simulink model "DC_current_phasor"  (R2016a)
settings: Solver=ode23t  StartTime=0.0  StopTime=2  MaxStep=1e-4  RelTol=1e-4  AbsTol=1e-4
undefined symbols (not defined in the file or in its folder): j, P
libraries: fl_lib x8, nesl_utility x8, pe_lib x3, ThreePhaseExamples_lib x1
Description:
  | Three-Phase Custom PMSM
  | 
  | This example shows a custom Simscape(TM) implementation of
  | a Permanent Magnet Synchronous Machine (PMSM). To view the
  | PMSM source code, double-click on the motor block and then
  | click on the hyperlink 'Source code'. This test circuit shows the
  | PMSM being used as a generator, the rectifier block converting
  | the induced AC back EMFs to a DC voltage which is in turn
  | applied to a resistive load.
  | 
  | 
  | 
  | Copyright 2008-2016 The MathWorks, Inc.
settings Model: Creator=MathWorks  LastModifiedBy=hbjo
settings DataIOCC: LimitDataPoints=on  SaveFormat=Array
settings DebuggingCC: UnderspecifiedInitializationDetection=Classic  MergeDetectMultiDrivingBlocksExec=none
settings HardwareCC: ProdBitPerPointer=32  ProdLargestAtomicFloat=None  ProdIntDivRoundTo=Undefined  ProdEndianess=Unspecified  ProdWordSize=32  ProdHWDeviceType=32-bit Generic
settings ModelReferenceCC: PropagateSignalLabelsOutOfModel=off
settings ConfigComp: CovModelRefEnable=Off  CovSFcnEnable=off
settings SimscapeCC: SimscapeLogDataHistory=50000

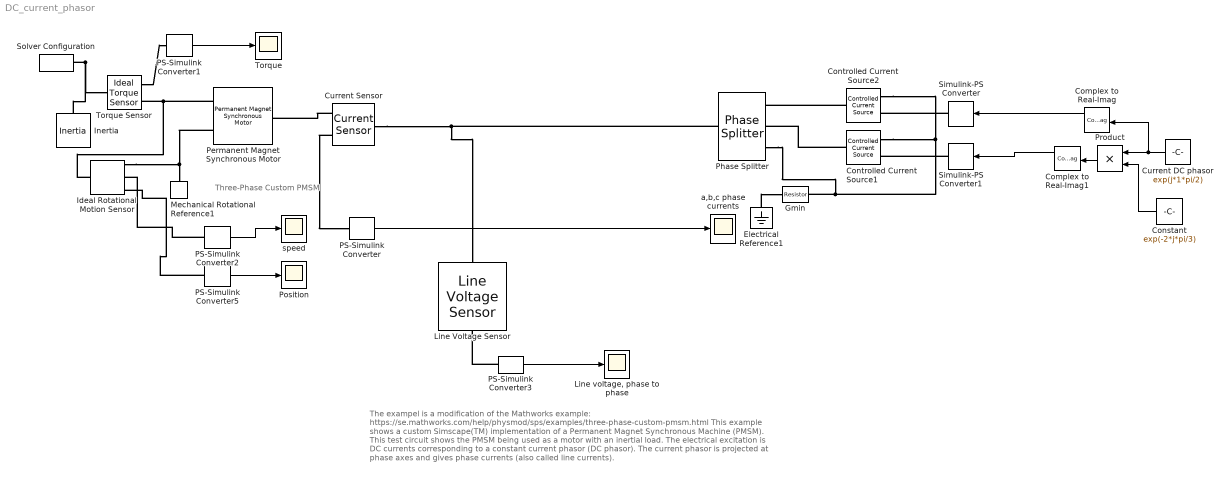
== system DC_current_phasor ==
  note: The exampel is a modification of the Mathworks example: https://se.mathworks.com/help/physmod/sps/examples/three-phase-custom-pmsm.html
      | This example shows a custom Simscape(TM) implementation of a Permanent Magnet Synchronous Machine (PMSM).
      | This test circuit shows the PMSM being used as a motor with an inertial load.
      | The electrical excitation is DC currents corresponding to a constant current phasor (DC phasor).
      | The current phasor is projected at phase axes and gives phase currents (also called line currents).
  note: Three-Phase Custom PMSM
  Complex to Real-Imag : ComplexToRealImag
  Complex to Real-Imag1 : ComplexToRealImag
  Constant : Constant  Value=exp(-2*j*pi/3)
  Controlled Current Source1 : fl_lib/Electrical/Electrical Sources/Controlled Current Source
  Controlled Current Source2 : fl_lib/Electrical/Electrical Sources/Controlled Current Source
  Current DC phasor : Constant  Value=exp(j*1*pi/2)
  Current Sensor : pe_lib/Sensors/Current Sensor
  Electrical Reference1 : fl_lib/Electrical/Electrical Elements/Electrical Reference
  Gmin : fl_lib/Electrical/Electrical Elements/Resistor  R=1e9 Ohm  i_specify=off  i_priority=High  i=0 A  v_specify=off  v_priority=High  v=0 V
  Ideal Rotational Motion Sensor : fl_lib/Mechanical/Mechanical Sensors/Ideal Rotational Motion Sensor  offset=0 rad
  Inertia : fl_lib/Mechanical/Rotational Elements/Inertia  inertia=0.005 kg*m^2  w_specify=off  w_priority=High  w=0 rad/s  t_specify=off  t_priority=None  t=0 N*m
  Line Voltage Sensor : pe_lib/Sensors/Line Voltage Sensor
  "Line voltage, phase to phase" : Scope
  Mechanical Rotational Reference1 : fl_lib/Mechanical/Rotational Elements/Mechanical Rotational Reference
  PS-Simulink Converter : nesl_utility/PS-Simulink Converter  PhysicalDomain=network_engine_domain  SubClassName=ps_output  LeftPortType=input  RightPortType=output  PseudoPeriodic=off  Frequencies=[]  Unit=A  AffineConversion=off
  PS-Simulink Converter1 : nesl_utility/PS-Simulink Converter  PhysicalDomain=network_engine_domain  SubClassName=ps_output  LeftPortType=input  RightPortType=output  PseudoPeriodic=off  Frequencies=[]  Unit=N*m  AffineConversion=off
  PS-Simulink Converter2 : nesl_utility/PS-Simulink Converter  PhysicalDomain=network_engine_domain  SubClassName=ps_output  LeftPortType=input  RightPortType=output  PseudoPeriodic=off  Frequencies=[]  Unit=rad/s  AffineConversion=off
  PS-Simulink Converter3 : nesl_utility/PS-Simulink Converter  PhysicalDomain=network_engine_domain  SubClassName=ps_output  LeftPortType=input  RightPortType=output  PseudoPeriodic=off  Frequencies=[]  Unit=V  AffineConversion=off
  PS-Simulink Converter5 : nesl_utility/PS-Simulink Converter  PhysicalDomain=network_engine_domain  SubClassName=ps_output  LeftPortType=input  RightPortType=output  PseudoPeriodic=off  Frequencies=[]  Unit=rad  AffineConversion=off
  Permanent Magnet Synchronous Motor : ThreePhaseExamples_lib/Permanent Magnet Synchronous Motor  nPolePairs=P/2  pm_flux_linkage=psi Wb  Ld=L H  Lq=L H  Rs=R Ohm  wNominal=0 rad/s  angular_position_diff_specify=off  angular_position_diff_priority=None  angular_position_diff=0 rad  i_d_specify=off  i_d_priority=High  i_d=0 A  i_q_specify=off  i_q_priority=High  i_q=0 A
  Phase Splitter : pe_lib/Connections/Phase Splitter
  Position : Scope
  Product : Product
  Simulink-PS Converter : nesl_utility/Simulink-PS Converter  PhysicalDomain=network_engine_domain  SubClassName=ps_input  LeftPortType=input  RightPortType=output  PseudoPeriodic=off  Frequencies=[]  NoiseDistribution=none  NoiseParameters=[]  Unit=1  AffineConversion=off  InputFiltering=off  SimscapeFilterOrder=1  InputFilterTimeConstant=0.001  UdotUserProvided=1
  Simulink-PS Converter1 : nesl_utility/Simulink-PS Converter  PhysicalDomain=network_engine_domain  SubClassName=ps_input  LeftPortType=input  RightPortType=output  PseudoPeriodic=off  Frequencies=[]  NoiseDistribution=none  NoiseParameters=[]  Unit=1  AffineConversion=off  InputFiltering=off  SimscapeFilterOrder=1  InputFilterTimeConstant=0.001  UdotUserProvided=1
  Solver Configuration : nesl_utility/Solver Configuration  PhysicalDomain=network_engine_domain  SubClassName=solver  LeftPortType=input  RightPortType=generic  Accelerate=off  Tones=[]  Harmonics=[]  SimulateNoise=off  Profile=off  UseLocalSampling=off  EnableSwitchedLinearOptims=on  FrequencyDomain=off  UseCCode=off  RelTol=0.001  AbsTol=1e-06  MinStep=1e-09  ToWorkspace=off  RevertToSquareIcSolve=off  NumHomotopyIterations=100  PhasorMode=off  PhasorModeNumHarmonics=1  OverrideAbsTol=off  DoDC=off  ResidualTolerance=1e-9  UseLocalSolver=on  LocalSolverChoice=NE_BACKWARD_EULER_ADVANCER  LocalSolverSampleTime=1e-5  DoFixedCost=on  MaxNonlinIter=3  MaxModeIter=2  LinearAlgebra=Sparse  DelaysMemoryBudget=1024  AutomaticFiltering=on  FilteringTimeConstant=0.001
  Torque : Scope
  Torque Sensor : fl_lib/Mechanical/Mechanical Sensors/Ideal Torque Sensor
  a,b,c phase currents : Scope
  speed : Scope
  wires:
  PS-Simulink Converter1/1 -> Torque/1
  PS-Simulink Converter3/1 -> "Line voltage, phase to phase"/1
  PS-Simulink Converter2/1 -> speed/1
  PS-Simulink Converter5/1 -> Position/1
  Complex to Real-Imag1/1 -> Simulink-PS Converter1/1
  Complex to Real-Imag/1 -> Simulink-PS Converter/1
  Constant/1 -> Product/2
  Product/1 -> Complex to Real-Imag1/1
  Current DC phasor/1 -> Complex to Real-Imag/1, Product/1
  PS-Simulink Converter/1 -> a,b,c phase currents/1
  connections:
  Permanent Magnet Synchronous Motor/RConn2 -- Ideal Rotational Motion Sensor/RConn1 -- Mechanical Rotational Reference1/LConn1
  Current Sensor/RConn1 -- PS-Simulink Converter/LConn1
  Permanent Magnet Synchronous Motor/RConn1 -- Ideal Rotational Motion Sensor/LConn1 -- Torque Sensor/RConn1
  Solver Configuration/RConn1 -- Inertia/LConn1 -- Torque Sensor/LConn1
  Electrical Reference1/LConn1 -- Gmin/LConn1
  PS-Simulink Converter3/LConn1 -- Line Voltage Sensor/RConn1
  Torque Sensor/RConn2 -- PS-Simulink Converter1/LConn1
  Phase Splitter/LConn1 -- Current Sensor/LConn1 -- Line Voltage Sensor/LConn1
  Controlled Current Source2/LConn1 -- Phase Splitter/RConn1
  Controlled Current Source1/LConn1 -- Phase Splitter/RConn2
  Controlled Current Source2/RConn2 -- Phase Splitter/RConn3 -- Gmin/RConn1 -- Controlled Current Source1/RConn2
  PS-Simulink Converter2/LConn1 -- Ideal Rotational Motion Sensor/RConn2
  PS-Simulink Converter5/LConn1 -- Ideal Rotational Motion Sensor/RConn3
  Simulink-PS Converter/RConn1 -- Controlled Current Source2/RConn1
  Simulink-PS Converter1/RConn1 -- Controlled Current Source1/RConn1
  Current Sensor/RConn2 -- Permanent Magnet Synchronous Motor/LConn1
